simulink model "case8"  (R2024b)
settings: Solver=FixedStepAuto  StartTime=0  StopTime=1  FixedStep=1e-7  RelTol=1e-3
values from neighbouring files (symbols this model uses):
  SG_D_1_D = 0.01056    [IEEE9_case_parameters.m]    (also in case1_parameters.m; case2_parameters.m; case3_parameters.m; case4_parameters.m)
  SG_D_1_EnableSaturation = 0    [IEEE9_case_parameters.m]    (also in case1_parameters.m; case2_parameters.m; case3_parameters.m; case4_parameters.m)
  SG_D_1_f0 = 60    [IEEE9_case_parameters.m]    (also in case1_parameters.m; case2_parameters.m; case3_parameters.m; case4_parameters.m)
  SG_D_1_H = 7.5    [IEEE9_case_parameters.m]    (also in case1_parameters.m; case2_parameters.m; case3_parameters.m; case4_parameters.m)
  SG_D_1_K_A = 20    [IEEE9_case_parameters.m]    (also in case1_parameters.m; case2_parameters.m; case3_parameters.m; case4_parameters.m)
  SG_D_1_K_E = 1.000000e+1    (= 10)    [IEEE9_case_parameters.m]    (also in case1_parameters.m; case2_parameters.m; case3_parameters.m; case4_parameters.m)
  SG_D_1_K_F = 2.363    [IEEE9_case_parameters.m]    (also in case1_parameters.m; case2_parameters.m; case3_parameters.m; case4_parameters.m)
  SG_D_1_K_s = 0.5    [IEEE9_case_parameters.m]    (also in case1_parameters.m = 5; case2_parameters.m = 5; case3_parameters.m = 5; case4_parameters.m = 5)
  SG_D_1_R_a = 0.001088    [IEEE9_case_parameters.m]    (also in case1_parameters.m; case2_parameters.m; case3_parameters.m; case4_parameters.m)
  SG_D_1_S_A = 1    [IEEE9_case_parameters.m]    (also in case1_parameters.m; case2_parameters.m; case3_parameters.m; case4_parameters.m)
  SG_D_1_S_B = 0.103    [IEEE9_case_parameters.m]    (also in case1_parameters.m; case2_parameters.m; case3_parameters.m; case4_parameters.m)
  SG_D_1_S_N = 10.659857    [IEEE9_case_parameters.m]    (also in case1_parameters.m; case2_parameters.m; case3_parameters.m; case4_parameters.m)
  SG_D_1_SpeedPara = 200    [IEEE9_case_parameters.m]    (also in case1_parameters.m; case2_parameters.m; case3_parameters.m; case4_parameters.m)
  SG_D_1_T_0 = 0.720173    [IEEE9_case_parameters.m]    (also in case1_parameters.m = 0.755522; case2_parameters.m = 0.808931; case3_parameters.m = 0.869402; case4_parameters.m = 0.729316)
  SG_D_1_T_1 = 0.3    [IEEE9_case_parameters.m]    (also in case1_parameters.m; case2_parameters.m; case3_parameters.m; case4_parameters.m)
  SG_D_1_T_2 = 0.05    [IEEE9_case_parameters.m]    (also in case1_parameters.m; case2_parameters.m; case3_parameters.m; case4_parameters.m)
  SG_D_1_T_3 = 0.02    [IEEE9_case_parameters.m]    (also in case1_parameters.m; case2_parameters.m; case3_parameters.m; case4_parameters.m)
  SG_D_1_T_4 = 0.005    [IEEE9_case_parameters.m]    (also in case1_parameters.m; case2_parameters.m; case3_parameters.m; case4_parameters.m)
  SG_D_1_T_A = 0.02    [IEEE9_case_parameters.m]    (also in case1_parameters.m; case2_parameters.m; case3_parameters.m; case4_parameters.m)
  SG_D_1_T_dd = 8.000000e+0    (= 8)    [IEEE9_case_parameters.m]    (also in case1_parameters.m; case2_parameters.m; case3_parameters.m; case4_parameters.m)
  SG_D_1_T_ddd = 0.04    [IEEE9_case_parameters.m]    (also in case1_parameters.m; case2_parameters.m; case3_parameters.m; case4_parameters.m)
  SG_D_1_T_E = 0.314    [IEEE9_case_parameters.m]    (also in case1_parameters.m; case2_parameters.m; case3_parameters.m; case4_parameters.m)
  SG_D_1_T_F = 0.35    [IEEE9_case_parameters.m]    (also in case1_parameters.m; case2_parameters.m; case3_parameters.m; case4_parameters.m)
  SG_D_1_T_qd = 0.8    [IEEE9_case_parameters.m]    (also in case1_parameters.m; case2_parameters.m; case3_parameters.m; case4_parameters.m)
  SG_D_1_T_qdd = 0.02    [IEEE9_case_parameters.m]    (also in case1_parameters.m; case2_parameters.m; case3_parameters.m; case4_parameters.m)
  SG_D_1_T_speed = 0.1    [IEEE9_case_parameters.m]    (also in case1_parameters.m = 200; case2_parameters.m = 200; case3_parameters.m = 200; case4_parameters.m = 200)
  SG_D_1_T_w = 0.5    [IEEE9_case_parameters.m]    (also in case1_parameters.m; case2_parameters.m; case3_parameters.m; case4_parameters.m)
  SG_D_1_V_ref = 1.990276    [IEEE9_case_parameters.m]    (also in case1_parameters.m = 2.042296; case2_parameters.m = 2.051388; case3_parameters.m = 2.089584; case4_parameters.m = 2.01845)
  SG_D_1_w_ref = 376.991118    [IEEE9_case_parameters.m]    (also in case1_parameters.m; case2_parameters.m; case3_parameters.m; case4_parameters.m)
  SG_D_1_wb = 6.000000e+1    (= 60)    [IEEE9_case_parameters.m]    (also in case1_parameters.m; case2_parameters.m; case3_parameters.m; case4_parameters.m)
  SG_D_1_x_d = 1.9    [IEEE9_case_parameters.m]    (also in case1_parameters.m; case2_parameters.m; case3_parameters.m; case4_parameters.m)
  SG_D_1_x_dd = 0.302    [IEEE9_case_parameters.m]    (also in case1_parameters.m; case2_parameters.m; case3_parameters.m; case4_parameters.m)
  SG_D_1_x_ddd = 0.204    [IEEE9_case_parameters.m]    (also in case1_parameters.m; case2_parameters.m; case3_parameters.m; case4_parameters.m)
  SG_D_1_x_l = 0.05    [IEEE9_case_parameters.m]    (also in case1_parameters.m; case2_parameters.m; case3_parameters.m; case4_parameters.m)
  SG_D_1_x_q = 1.3    [IEEE9_case_parameters.m]    (also in case1_parameters.m; case2_parameters.m; case3_parameters.m; case4_parameters.m)
  SG_D_1_x_qd = 0.5    [IEEE9_case_parameters.m]    (also in case1_parameters.m; case2_parameters.m; case3_parameters.m; case4_parameters.m)
  SG_D_1_x_qdd = 0.3    [IEEE9_case_parameters.m]    (also in case1_parameters.m; case2_parameters.m; case3_parameters.m; case4_parameters.m)
  SG_D_2_D = 0.02    [IEEE9_case_parameters.m]    (also in case1_parameters.m; case2_parameters.m; case3_parameters.m; case4_parameters.m)
  SG_D_2_EnableSaturation = 0    [IEEE9_case_parameters.m]    (also in case1_parameters.m; case2_parameters.m; case3_parameters.m; case4_parameters.m)
  SG_D_2_f0 = 60    [IEEE9_case_parameters.m]    (also in case1_parameters.m; case2_parameters.m; case3_parameters.m; case4_parameters.m)
  SG_D_2_H = 8.000000e+0    (= 8)    [IEEE9_case_parameters.m]    (also in case1_parameters.m; case2_parameters.m; case3_parameters.m; case4_parameters.m)
  SG_D_2_K_A = 20    [IEEE9_case_parameters.m]    (also in case1_parameters.m; case2_parameters.m; case3_parameters.m; case4_parameters.m)
  SG_D_2_K_E = 1.000000e+1    (= 10)    [IEEE9_case_parameters.m]    (also in case1_parameters.m; case2_parameters.m; case3_parameters.m; case4_parameters.m)
  SG_D_2_K_F = 2.363    [IEEE9_case_parameters.m]    (also in case1_parameters.m; case2_parameters.m; case3_parameters.m; case4_parameters.m)
  SG_D_2_K_s = 0.5    [IEEE9_case_parameters.m]    (also in case1_parameters.m = 4; case2_parameters.m = 4; case3_parameters.m = 4; case4_parameters.m = 4)
  SG_D_2_R_a = 0.001088    [IEEE9_case_parameters.m]    (also in case1_parameters.m; case2_parameters.m; case3_parameters.m; case4_parameters.m)
  SG_D_2_S_A = 1    [IEEE9_case_parameters.m]    (also in case1_parameters.m; case2_parameters.m; case3_parameters.m; case4_parameters.m)
  SG_D_2_S_B = 0.103    [IEEE9_case_parameters.m]    (also in case1_parameters.m; case2_parameters.m; case3_parameters.m; case4_parameters.m)
  SG_D_2_S_N = 10.659857    [IEEE9_case_parameters.m]    (also in case1_parameters.m; case2_parameters.m; case3_parameters.m; case4_parameters.m)
  SG_D_2_SpeedPara = 200    [IEEE9_case_parameters.m]    (also in case1_parameters.m; case2_parameters.m; case3_parameters.m; case4_parameters.m)
  SG_D_2_T_0 = 1.632913    [IEEE9_case_parameters.m]    (also in case1_parameters.m = 1.632925; case2_parameters.m = 1.632915; case3_parameters.m = 1.632914; case4_parameters.m = 1.632927)
  SG_D_2_T_1 = 0.2    [IEEE9_case_parameters.m]    (also in case1_parameters.m; case2_parameters.m; case3_parameters.m; case4_parameters.m)
  SG_D_2_T_2 = 0.05    [IEEE9_case_parameters.m]    (also in case1_parameters.m; case2_parameters.m; case3_parameters.m; case4_parameters.m)
  SG_D_2_T_3 = 0.02    [IEEE9_case_parameters.m]    (also in case1_parameters.m; case2_parameters.m; case3_parameters.m; case4_parameters.m)
  SG_D_2_T_4 = 0.005    [IEEE9_case_parameters.m]    (also in case1_parameters.m; case2_parameters.m; case3_parameters.m; case4_parameters.m)
  SG_D_2_T_A = 0.02    [IEEE9_case_parameters.m]    (also in case1_parameters.m; case2_parameters.m; case3_parameters.m; case4_parameters.m)
  SG_D_2_T_dd = 7.9    [IEEE9_case_parameters.m]    (also in case1_parameters.m; case2_parameters.m; case3_parameters.m; case4_parameters.m)
  SG_D_2_T_ddd = 0.04    [IEEE9_case_parameters.m]    (also in case1_parameters.m; case2_parameters.m; case3_parameters.m; case4_parameters.m)
  SG_D_2_T_E = 0.314    [IEEE9_case_parameters.m]    (also in case1_parameters.m; case2_parameters.m; case3_parameters.m; case4_parameters.m)
  SG_D_2_T_F = 0.35    [IEEE9_case_parameters.m]    (also in case1_parameters.m; case2_parameters.m; case3_parameters.m; case4_parameters.m)
  SG_D_2_T_qd = 0.8    [IEEE9_case_parameters.m]    (also in case1_parameters.m; case2_parameters.m; case3_parameters.m; case4_parameters.m)
  SG_D_2_T_qdd = 0.015    [IEEE9_case_parameters.m]    (also in case1_parameters.m; case2_parameters.m; case3_parameters.m; case4_parameters.m)
  SG_D_2_T_speed = 0.1    [IEEE9_case_parameters.m]    (also in case1_parameters.m = 150; case2_parameters.m = 150; case3_parameters.m = 150; case4_parameters.m = 150)
  SG_D_2_T_w = 0.35    [IEEE9_case_parameters.m]    (also in case1_parameters.m; case2_parameters.m; case3_parameters.m; case4_parameters.m)
  SG_D_2_V_ref = 2.58547    [IEEE9_case_parameters.m]    (also in case1_parameters.m = 2.597896; case2_parameters.m = 2.587136; case3_parameters.m = 2.586042; case4_parameters.m = 2.599679)
  SG_D_2_w_ref = 376.991118    [IEEE9_case_parameters.m]    (also in case1_parameters.m; case2_parameters.m; case3_parameters.m; case4_parameters.m)
  SG_D_2_wb = 6.000000e+1    (= 60)    [IEEE9_case_parameters.m]    (also in case1_parameters.m; case2_parameters.m; case3_parameters.m; case4_parameters.m)
  SG_D_2_x_d = 1.8    [IEEE9_case_parameters.m]    (also in case1_parameters.m; case2_parameters.m; case3_parameters.m; case4_parameters.m)
  SG_D_2_x_dd = 0.302    [IEEE9_case_parameters.m]    (also in case1_parameters.m; case2_parameters.m; case3_parameters.m; case4_parameters.m)
  SG_D_2_x_ddd = 0.204    [IEEE9_case_parameters.m]    (also in case1_parameters.m; case2_parameters.m; case3_parameters.m; case4_parameters.m)
  SG_D_2_x_l = 0.05    [IEEE9_case_parameters.m]    (also in case1_parameters.m; case2_parameters.m; case3_parameters.m; case4_parameters.m)
  SG_D_2_x_q = 1.25    [IEEE9_case_parameters.m]    (also in case1_parameters.m; case2_parameters.m; case3_parameters.m; case4_parameters.m)
  SG_D_2_x_qd = 0.5    [IEEE9_case_parameters.m]    (also in case1_parameters.m; case2_parameters.m; case3_parameters.m; case4_parameters.m)
  SG_D_2_x_qdd = 0.3    [IEEE9_case_parameters.m]    (also in case1_parameters.m; case2_parameters.m; case3_parameters.m; case4_parameters.m)
  SG_D_3_D = 0.02    [IEEE9_case_parameters.m]    (also in case1_parameters.m; case2_parameters.m; case3_parameters.m; case4_parameters.m)
  SG_D_3_EnableSaturation = 0    [IEEE9_case_parameters.m]    (also in case1_parameters.m; case2_parameters.m; case3_parameters.m; case4_parameters.m)
  SG_D_3_f0 = 60    [IEEE9_case_parameters.m]    (also in case1_parameters.m; case2_parameters.m; case3_parameters.m; case4_parameters.m)
  SG_D_3_H = 7.7    [IEEE9_case_parameters.m]    (also in case1_parameters.m; case2_parameters.m; case3_parameters.m; case4_parameters.m)
  SG_D_3_K_A = 20    [IEEE9_case_parameters.m]    (also in case1_parameters.m; case2_parameters.m; case3_parameters.m; case4_parameters.m)
  SG_D_3_K_E = 1.000000e+1    (= 10)    [IEEE9_case_parameters.m]    (also in case1_parameters.m; case2_parameters.m; case3_parameters.m; case4_parameters.m)
  SG_D_3_K_F = 2.363    [IEEE9_case_parameters.m]    (also in case1_parameters.m; case2_parameters.m; case3_parameters.m; case4_parameters.m)
  SG_D_3_K_s = 0.2    [IEEE9_case_parameters.m]    (also in case1_parameters.m = 2; case2_parameters.m = 2; case3_parameters.m = 2; case4_parameters.m = 2)
  SG_D_3_R_a = 0.001088    [IEEE9_case_parameters.m]    (also in case1_parameters.m; case2_parameters.m; case3_parameters.m; case4_parameters.m)
  SG_D_3_S_A = 1    [IEEE9_case_parameters.m]    (also in case1_parameters.m; case2_parameters.m; case3_parameters.m; case4_parameters.m)
  SG_D_3_S_B = 0.103    [IEEE9_case_parameters.m]    (also in case1_parameters.m; case2_parameters.m; case3_parameters.m; case4_parameters.m)
  SG_D_3_S_N = 10.659857    [IEEE9_case_parameters.m]    (also in case1_parameters.m; case2_parameters.m; case3_parameters.m; case4_parameters.m)
  SG_D_3_SpeedPara = 200    [IEEE9_case_parameters.m]    (also in case1_parameters.m; case2_parameters.m; case3_parameters.m; case4_parameters.m)
  SG_D_3_T_0 = 0.850788    [IEEE9_case_parameters.m]    (also in case1_parameters.m = 0.850786; case2_parameters.m = 0.850787; case3_parameters.m; case4_parameters.m = 0.850786)
  SG_D_3_T_1 = 0.2    [IEEE9_case_parameters.m]    (also in case1_parameters.m; case2_parameters.m; case3_parameters.m; case4_parameters.m)
  SG_D_3_T_2 = 0.05    [IEEE9_case_parameters.m]    (also in case1_parameters.m; case2_parameters.m; case3_parameters.m; case4_parameters.m)
  SG_D_3_T_3 = 0.02    [IEEE9_case_parameters.m]    (also in case1_parameters.m; case2_parameters.m; case3_parameters.m; case4_parameters.m)
  SG_D_3_T_4 = 0.005    [IEEE9_case_parameters.m]    (also in case1_parameters.m; case2_parameters.m; case3_parameters.m; case4_parameters.m)
  SG_D_3_T_A = 0.02    [IEEE9_case_parameters.m]    (also in case1_parameters.m; case2_parameters.m; case3_parameters.m; case4_parameters.m)
  SG_D_3_T_dd = 8.1    [IEEE9_case_parameters.m]    (also in case1_parameters.m; case2_parameters.m; case3_parameters.m; case4_parameters.m)
  SG_D_3_T_ddd = 0.04    [IEEE9_case_parameters.m]    (also in case1_parameters.m; case2_parameters.m; case3_parameters.m; case4_parameters.m)
  SG_D_3_T_E = 0.314    [IEEE9_case_parameters.m]    (also in case1_parameters.m; case2_parameters.m; case3_parameters.m; case4_parameters.m)
  SG_D_3_T_F = 0.35    [IEEE9_case_parameters.m]    (also in case1_parameters.m; case2_parameters.m; case3_parameters.m; case4_parameters.m)
  SG_D_3_T_qd = 0.8    [IEEE9_case_parameters.m]    (also in case1_parameters.m; case2_parameters.m; case3_parameters.m; case4_parameters.m)
  SG_D_3_T_qdd = 0.015    [IEEE9_case_parameters.m]    (also in case1_parameters.m; case2_parameters.m; case3_parameters.m; case4_parameters.m)
  SG_D_3_T_speed = 0.1    [IEEE9_case_parameters.m]    (also in case1_parameters.m = 180; case2_parameters.m = 180; case3_parameters.m = 180; case4_parameters.m = 180)
  SG_D_3_T_w = 0.4    [IEEE9_case_parameters.m]    (also in case1_parameters.m; case2_parameters.m; case3_parameters.m; case4_parameters.m)
  SG_D_3_V_ref = 1.892727    [IEEE9_case_parameters.m]    (also in case1_parameters.m = 1.906439; case2_parameters.m = 1.895535; case3_parameters.m = 1.892105; case4_parameters.m = 1.906598)
  SG_D_3_w_ref = 376.991118    [IEEE9_case_parameters.m]    (also in case1_parameters.m; case2_parameters.m; case3_parameters.m; case4_parameters.m)
  SG_D_3_wb = 6.000000e+1    (= 60)    [IEEE9_case_parameters.m]    (also in case1_parameters.m; case2_parameters.m; case3_parameters.m; case4_parameters.m)
  SG_D_3_x_d = 1.85    [IEEE9_case_parameters.m]    (also in case1_parameters.m; case2_parameters.m; case3_parameters.m; case4_parameters.m)
  SG_D_3_x_dd = 0.302    [IEEE9_case_parameters.m]    (also in case1_parameters.m; case2_parameters.m; case3_parameters.m; case4_parameters.m)
  SG_D_3_x_ddd = 0.204    [IEEE9_case_parameters.m]    (also in case1_parameters.m; case2_parameters.m; case3_parameters.m; case4_parameters.m)
  SG_D_3_x_l = 0.05    [IEEE9_case_parameters.m]    (also in case1_parameters.m; case2_parameters.m; case3_parameters.m; case4_parameters.m)
  SG_D_3_x_q = 1.2    [IEEE9_case_parameters.m]    (also in case1_parameters.m; case2_parameters.m; case3_parameters.m; case4_parameters.m)
  SG_D_3_x_qd = 0.5    [IEEE9_case_parameters.m]    (also in case1_parameters.m; case2_parameters.m; case3_parameters.m; case4_parameters.m)
  SG_D_3_x_qdd = 0.3    [IEEE9_case_parameters.m]    (also in case1_parameters.m; case2_parameters.m; case3_parameters.m; case4_parameters.m)
(part 2 of 12)

== system case8/SG_D_2 ==
  v_d_SG_D_2 : Inport
  v_q_SG_D_2 : Inport  Port=2
  E_fd_SG_D_2 : Integrator  InitialCondition=3.1461551283845077
  Px_1_SG_D_2 : Integrator  InitialCondition=0.0
  Px_2_SG_D_2 : Integrator  InitialCondition=0.0
  Px_3_SG_D_2 : Integrator  InitialCondition=-1.4463668526796511e-25
  R_f_SG_D_2 : Integrator  InitialCondition=21.241041623921692
  T_e_SG_D_2_block : Subsystem
  T_m_SG_D_2 : Integrator  InitialCondition=1.6329038289025481
  V_f_SG_D_2 : Integrator  InitialCondition=31.46155128384508
  d_E_fd_SG_D_2_block : Subsystem
  d_Px_1_SG_D_2_block : Subsystem
  d_Px_2_SG_D_2_block : Subsystem
  d_Px_3_SG_D_2_block : Subsystem
  d_R_f_SG_D_2_block : Subsystem
  d_T_m_SG_D_2_block : Subsystem
  d_V_f_SG_D_2_block : Subsystem
  d_psi_1d_SG_D_2_block : Subsystem
  d_psi_d_SG_D_2_block : Subsystem
  d_psi_fd_SG_D_2_block : Subsystem
  d_psi_gq_SG_D_2_block : Subsystem
  d_psi_kq_SG_D_2_block : Subsystem
  d_psi_q_SG_D_2_block : Subsystem
  d_theta_SG_D_2_block : Subsystem
  d_w_SG_D_2_block : Subsystem
  i_d_SG_D_2_block : Subsystem
  i_q_SG_D_2_block : Subsystem
  psi_1d_SG_D_2 : Integrator  InitialCondition=0.5625664495240386
  psi_d_SG_D_2 : Integrator  InitialCondition=0.4887496301280251
  psi_fd_SG_D_2 : Integrator  InitialCondition=0.9346032192799462
  psi_gq_SG_D_2 : Integrator  InitialCondition=0.524673786109037
  psi_kq_SG_D_2 : Integrator  InitialCondition=-0.8394780577744592
  psi_q_SG_D_2 : Integrator  InitialCondition=-0.8744563101817284
  theta_SG_D_2 : Integrator  InitialCondition=1.2359602856549958
  theta_SG_D_2_out_block : Subsystem
  w_SG_D_2 : Integrator  InitialCondition=376.99111843077515
  w_SG_D_2_out_block : Subsystem
  i_d_SG_D_2 : Outport
  i_q_SG_D_2 : Outport  Port=2
  T_e_SG_D_2 : Outport  Port=3
  w_SG_D_2_out : Outport  Port=4
  theta_SG_D_2_out : Outport  Port=5
  wires:
  T_e_SG_D_2_block/1(Blockout_T_e_SG_D_2_37eed) -> T_e_SG_D_2/1
  d_Px_2_SG_D_2_block/1(Blockout_d_Px_2_SG_D_2_834a7) -> Px_2_SG_D_2/1
  d_T_m_SG_D_2_block/1(Blockout_d_T_m_SG_D_2_9d432) -> T_m_SG_D_2/1
  w_SG_D_2/1 -> d_psi_d_SG_D_2_block/9(State_w_SG_D_2_45274), d_psi_q_SG_D_2_block/9(State_w_SG_D_2_341ca), d_w_SG_D_2_block/1(State_w_SG_D_2_ba66f), d_V_f_SG_D_2_block/8(State_w_SG_D_2_40010), d_V_f_SG_D_2_block/13(State_w_SG_D_2_e6aa6), d_T_m_SG_D_2_block/1(State_w_SG_D_2_f6fcd), d_Px_1_SG_D_2_block/2(State_w_SG_D_2_e8896), d_Px_2_SG_D_2_block/4(State_w_SG_D_2_770a4), d_theta_SG_D_2_block/1(State_w_SG_D_2_7bd31), d_Px_3_SG_D_2_block/6(State_w_SG_D_2_e0f2c), w_SG_D_2_out_block/1(State_w_SG_D_2_c1838)
  psi_fd_SG_D_2/1 -> d_psi_fd_SG_D_2_block/4(State_psi_fd_SG_D_2_4158a), d_psi_fd_SG_D_2_block/2(State_psi_fd_SG_D_2_b4c0c), d_psi_fd_SG_D_2_block/7(State_psi_fd_SG_D_2_07a98), d_psi_fd_SG_D_2_block/10(State_psi_fd_SG_D_2_1b762), d_psi_d_SG_D_2_block/3(State_psi_fd_SG_D_2_72f19), d_psi_1d_SG_D_2_block/2(State_psi_fd_SG_D_2_ceb12), d_psi_1d_SG_D_2_block/5(State_psi_fd_SG_D_2_a1da1), i_d_SG_D_2_block/7(State_psi_fd_SG_D_2_bfe7a), i_q_SG_D_2_block/7(State_psi_fd_SG_D_2_88a91), d_w_SG_D_2_block/10(State_psi_fd_SG_D_2_18877), d_V_f_SG_D_2_block/6(State_psi_fd_SG_D_2_2a738), T_e_SG_D_2_block/8(State_psi_fd_SG_D_2_89a99)
  d_Px_3_SG_D_2_block/1(Blockout_d_Px_3_SG_D_2_f4998) -> Px_3_SG_D_2/1
  d_theta_SG_D_2_block/1(Blockout_d_theta_SG_D_2_25192) -> theta_SG_D_2/1
  psi_q_SG_D_2/1 -> d_psi_d_SG_D_2_block/8(State_psi_q_SG_D_2_6ca96), d_psi_q_SG_D_2_block/3(State_psi_q_SG_D_2_4fbbc), d_psi_gq_SG_D_2_block/6(State_psi_q_SG_D_2_7c5c2), d_psi_gq_SG_D_2_block/9(State_psi_q_SG_D_2_071fc), d_psi_kq_SG_D_2_block/5(State_psi_q_SG_D_2_e3912), d_w_SG_D_2_block/6(State_psi_q_SG_D_2_719d4), d_V_f_SG_D_2_block/7(State_psi_q_SG_D_2_06b5a), d_w_SG_D_2_block/7(State_psi_q_SG_D_2_47440), d_V_f_SG_D_2_block/11(State_psi_q_SG_D_2_14190), T_e_SG_D_2_block/4(State_psi_q_SG_D_2_d1f35), i_d_SG_D_2_block/3(State_psi_q_SG_D_2_62810), T_e_SG_D_2_block/5(State_psi_q_SG_D_2_dcfde), i_q_SG_D_2_block/3(State_psi_q_SG_D_2_6a090)
  w_SG_D_2_out_block/1(Blockout_w_SG_D_2_out_5dbba) -> w_SG_D_2_out/1
  d_Px_1_SG_D_2_block/1(Blockout_d_Px_1_SG_D_2_3d98f) -> Px_1_SG_D_2/1
  theta_SG_D_2/1 -> d_psi_d_SG_D_2_block/5(State_theta_SG_D_2_93d8b), d_psi_d_SG_D_2_block/7(State_theta_SG_D_2_1c678), d_psi_q_SG_D_2_block/7(State_theta_SG_D_2_47452), i_d_SG_D_2_block/4(State_theta_SG_D_2_8321e), i_q_SG_D_2_block/4(State_theta_SG_D_2_61b92), i_q_SG_D_2_block/8(State_theta_SG_D_2_36c34), i_d_SG_D_2_block/8(State_theta_SG_D_2_8d67b), theta_SG_D_2_out_block/1(State_theta_SG_D_2_588b5), d_psi_q_SG_D_2_block/5(State_theta_SG_D_2_e72a3)
  v_d_SG_D_2/1 -> d_psi_d_SG_D_2_block/4(Input_v_d_SG_D_2_0b52f), d_psi_q_SG_D_2_block/4(Input_v_d_SG_D_2_d12f5)
  psi_gq_SG_D_2/1 -> d_psi_q_SG_D_2_block/1(State_psi_gq_SG_D_2_5ef83), d_psi_gq_SG_D_2_block/1(State_psi_gq_SG_D_2_6e627), d_psi_gq_SG_D_2_block/2(State_psi_gq_SG_D_2_262b6), d_psi_gq_SG_D_2_block/4(State_psi_gq_SG_D_2_5c0ba), d_psi_kq_SG_D_2_block/3(State_psi_gq_SG_D_2_5efea), d_w_SG_D_2_block/4(State_psi_gq_SG_D_2_4cbe9), d_psi_gq_SG_D_2_block/7(State_psi_gq_SG_D_2_708e2), d_V_f_SG_D_2_block/9(State_psi_gq_SG_D_2_0beb3), d_psi_kq_SG_D_2_block/1(State_psi_gq_SG_D_2_71331), T_e_SG_D_2_block/2(State_psi_gq_SG_D_2_6b895), i_q_SG_D_2_block/1(State_psi_gq_SG_D_2_ca4a4), i_d_SG_D_2_block/1(State_psi_gq_SG_D_2_6632a)
  d_V_f_SG_D_2_block/1(Blockout_d_V_f_SG_D_2_ff4c4) -> V_f_SG_D_2/1
  v_q_SG_D_2/1 -> d_psi_d_SG_D_2_block/6(Input_v_q_SG_D_2_24264), d_psi_q_SG_D_2_block/6(Input_v_q_SG_D_2_08eca)
  psi_kq_SG_D_2/1 -> d_psi_q_SG_D_2_block/2(State_psi_kq_SG_D_2_f0515), d_psi_gq_SG_D_2_block/3(State_psi_kq_SG_D_2_70141), d_psi_gq_SG_D_2_block/5(State_psi_kq_SG_D_2_f72a7), d_psi_gq_SG_D_2_block/8(State_psi_kq_SG_D_2_8a990), d_w_SG_D_2_block/5(State_psi_kq_SG_D_2_af1ac), d_V_f_SG_D_2_block/10(State_psi_kq_SG_D_2_49fef), d_psi_kq_SG_D_2_block/2(State_psi_kq_SG_D_2_cb04f), i_d_SG_D_2_block/2(State_psi_kq_SG_D_2_999f9), i_q_SG_D_2_block/2(State_psi_kq_SG_D_2_2a403), T_e_SG_D_2_block/3(State_psi_kq_SG_D_2_20085), d_psi_kq_SG_D_2_block/4(State_psi_kq_SG_D_2_ff070)
  i_d_SG_D_2_block/1(Blockout_i_d_SG_D_2_06834) -> i_d_SG_D_2/1
  psi_d_SG_D_2/1 -> d_psi_fd_SG_D_2_block/9(State_psi_d_SG_D_2_0ff1e), d_psi_q_SG_D_2_block/8(State_psi_d_SG_D_2_64c51), d_psi_1d_SG_D_2_block/4(State_psi_d_SG_D_2_bd43f), d_w_SG_D_2_block/3(State_psi_d_SG_D_2_74fc0), d_psi_d_SG_D_2_block/2(State_psi_d_SG_D_2_6f046), d_psi_fd_SG_D_2_block/6(State_psi_d_SG_D_2_db85c), d_w_SG_D_2_block/9(State_psi_d_SG_D_2_c6663), d_V_f_SG_D_2_block/12(State_psi_d_SG_D_2_55d30), d_V_f_SG_D_2_block/5(State_psi_d_SG_D_2_02653), i_d_SG_D_2_block/6(State_psi_d_SG_D_2_05ecc), i_q_SG_D_2_block/6(State_psi_d_SG_D_2_04a53), T_e_SG_D_2_block/1(State_psi_d_SG_D_2_f5fd7), T_e_SG_D_2_block/7(State_psi_d_SG_D_2_0c163)
  Px_1_SG_D_2/1 -> d_Px_1_SG_D_2_block/1(State_Px_1_SG_D_2_1fdac), d_Px_2_SG_D_2_block/3(State_Px_1_SG_D_2_2790d), d_Px_3_SG_D_2_block/4(State_Px_1_SG_D_2_7fb84), d_Px_3_SG_D_2_block/5(State_Px_1_SG_D_2_3fef0), d_Px_2_SG_D_2_block/2(State_Px_1_SG_D_2_d6347)
  T_m_SG_D_2/1 -> d_T_m_SG_D_2_block/2(State_T_m_SG_D_2_95b0e), d_w_SG_D_2_block/2(State_T_m_SG_D_2_44cee)
  Px_2_SG_D_2/1 -> d_Px_2_SG_D_2_block/1(State_Px_2_SG_D_2_8f0fc), d_Px_3_SG_D_2_block/2(State_Px_2_SG_D_2_e8830), d_Px_3_SG_D_2_block/3(State_Px_2_SG_D_2_b92ad)
  psi_1d_SG_D_2/1 -> d_psi_fd_SG_D_2_block/8(State_psi_1d_SG_D_2_d512d), d_psi_fd_SG_D_2_block/5(State_psi_1d_SG_D_2_923e8), d_psi_d_SG_D_2_block/1(State_psi_1d_SG_D_2_aad77), d_psi_fd_SG_D_2_block/3(State_psi_1d_SG_D_2_30ef8), d_psi_1d_SG_D_2_block/3(State_psi_1d_SG_D_2_f87fc), d_w_SG_D_2_block/8(State_psi_1d_SG_D_2_235de), d_psi_1d_SG_D_2_block/1(State_psi_1d_SG_D_2_34802), d_V_f_SG_D_2_block/4(State_psi_1d_SG_D_2_6ad6a), i_d_SG_D_2_block/5(State_psi_1d_SG_D_2_4ff2d), i_q_SG_D_2_block/5(State_psi_1d_SG_D_2_1de77), T_e_SG_D_2_block/6(State_psi_1d_SG_D_2_b2612)
  d_R_f_SG_D_2_block/1(Blockout_d_R_f_SG_D_2_8501b) -> R_f_SG_D_2/1
  d_psi_gq_SG_D_2_block/1(Blockout_d_psi_gq_SG_D_2_9dda3) -> psi_gq_SG_D_2/1
  d_psi_kq_SG_D_2_block/1(Blockout_d_psi_kq_SG_D_2_314e9) -> psi_kq_SG_D_2/1
  R_f_SG_D_2/1 -> d_V_f_SG_D_2_block/2(State_R_f_SG_D_2_4eb2e), d_R_f_SG_D_2_block/2(State_R_f_SG_D_2_76268)
  theta_SG_D_2_out_block/1(Blockout_theta_SG_D_2_out_80a64) -> theta_SG_D_2_out/1
  i_q_SG_D_2_block/1(Blockout_i_q_SG_D_2_51e7b) -> i_q_SG_D_2/1
  d_psi_q_SG_D_2_block/1(Blockout_d_psi_q_SG_D_2_ca292) -> psi_q_SG_D_2/1
  d_psi_d_SG_D_2_block/1(Blockout_d_psi_d_SG_D_2_41311) -> psi_d_SG_D_2/1
  d_w_SG_D_2_block/1(Blockout_d_w_SG_D_2_560c9) -> w_SG_D_2/1
  d_psi_1d_SG_D_2_block/1(Blockout_d_psi_1d_SG_D_2_8d877) -> psi_1d_SG_D_2/1
  V_f_SG_D_2/1 -> d_V_f_SG_D_2_block/14(State_V_f_SG_D_2_79586), d_E_fd_SG_D_2_block/2(State_V_f_SG_D_2_b3f2e)
  Px_3_SG_D_2/1 -> d_V_f_SG_D_2_block/3(State_Px_3_SG_D_2_61526), d_Px_3_SG_D_2_block/1(State_Px_3_SG_D_2_a00f9)
  d_E_fd_SG_D_2_block/1(Blockout_d_E_fd_SG_D_2_a4411) -> E_fd_SG_D_2/1
  E_fd_SG_D_2/1 -> d_R_f_SG_D_2_block/1(State_E_fd_SG_D_2_59077), d_V_f_SG_D_2_block/1(State_E_fd_SG_D_2_d52e1), d_E_fd_SG_D_2_block/1(State_E_fd_SG_D_2_423a9), d_psi_fd_SG_D_2_block/1(State_E_fd_SG_D_2_e61ef)
  d_psi_fd_SG_D_2_block/1(Blockout_d_psi_fd_SG_D_2_e5dbf) -> psi_fd_SG_D_2/1

== system case8/SG_D_3 ==
  v_d_SG_D_3 : Inport
  v_q_SG_D_3 : Inport  Port=2
  E_fd_SG_D_3 : Integrator  InitialCondition=1.7532139531153585
  Px_1_SG_D_3 : Integrator  InitialCondition=0.0
  Px_2_SG_D_3 : Integrator  InitialCondition=0.0
  Px_3_SG_D_3 : Integrator  InitialCondition=9.861433339358398e-25
  R_f_SG_D_3 : Integrator  InitialCondition=11.836698774890264
  T_e_SG_D_3_block : Subsystem
  T_m_SG_D_3 : Integrator  InitialCondition=0.8507912366770715
  V_f_SG_D_3 : Integrator  InitialCondition=17.532139531153582
  d_E_fd_SG_D_3_block : Subsystem
  d_Px_1_SG_D_3_block : Subsystem
  d_Px_2_SG_D_3_block : Subsystem
  d_Px_3_SG_D_3_block : Subsystem
  d_R_f_SG_D_3_block : Subsystem
  d_T_m_SG_D_3_block : Subsystem
  d_V_f_SG_D_3_block : Subsystem
  d_psi_1d_SG_D_3_block : Subsystem
  d_psi_d_SG_D_3_block : Subsystem
  d_psi_fd_SG_D_3_block : Subsystem
  d_psi_gq_SG_D_3_block : Subsystem
  d_psi_kq_SG_D_3_block : Subsystem
  d_psi_q_SG_D_3_block : Subsystem
  d_theta_SG_D_3_block : Subsystem
  d_w_SG_D_3_block : Subsystem
  i_d_SG_D_3_block : Subsystem
  i_q_SG_D_3_block : Subsystem
  psi_1d_SG_D_3 : Integrator  InitialCondition=0.6990200101655261
  psi_d_SG_D_3 : Integrator  InitialCondition=0.6697368450835861
  psi_fd_SG_D_3 : Integrator  InitialCondition=0.8466071621785026
  psi_gq_SG_D_3 : Integrator  InitialCondition=0.4339086560646932
  psi_kq_SG_D_3 : Integrator  InitialCondition=-0.7128499349634246
  psi_q_SG_D_3 : Integrator  InitialCondition=-0.7438434103966169
  theta_SG_D_3 : Integrator  InitialCondition=0.9265669299712972
  theta_SG_D_3_out_block : Subsystem
  w_SG_D_3 : Integrator  InitialCondition=376.99111843077515
  w_SG_D_3_out_block : Subsystem
  i_d_SG_D_3 : Outport
  i_q_SG_D_3 : Outport  Port=2
  T_e_SG_D_3 : Outport  Port=3
  w_SG_D_3_out : Outport  Port=4
  theta_SG_D_3_out : Outport  Port=5
  wires:
  psi_q_SG_D_3/1 -> d_psi_d_SG_D_3_block/8(State_psi_q_SG_D_3_c42a8), d_psi_q_SG_D_3_block/3(State_psi_q_SG_D_3_c2b51), d_psi_gq_SG_D_3_block/6(State_psi_q_SG_D_3_5b7d5), d_psi_gq_SG_D_3_block/9(State_psi_q_SG_D_3_a2ccc), d_psi_kq_SG_D_3_block/5(State_psi_q_SG_D_3_9bd31), d_w_SG_D_3_block/6(State_psi_q_SG_D_3_ce2ac), d_V_f_SG_D_3_block/7(State_psi_q_SG_D_3_86bf4), d_w_SG_D_3_block/7(State_psi_q_SG_D_3_ecc92), i_d_SG_D_3_block/3(State_psi_q_SG_D_3_5ee11), T_e_SG_D_3_block/4(State_psi_q_SG_D_3_35d7e), i_q_SG_D_3_block/3(State_psi_q_SG_D_3_862db), T_e_SG_D_3_block/5(State_psi_q_SG_D_3_c727a), d_V_f_SG_D_3_block/11(State_psi_q_SG_D_3_c4568)
  d_Px_1_SG_D_3_block/1(Blockout_d_Px_1_SG_D_3_077a4) -> Px_1_SG_D_3/1
  w_SG_D_3/1 -> d_psi_q_SG_D_3_block/9(State_w_SG_D_3_cea80), d_w_SG_D_3_block/1(State_w_SG_D_3_f0746), d_V_f_SG_D_3_block/13(State_w_SG_D_3_9dc31), d_V_f_SG_D_3_block/8(State_w_SG_D_3_db882), d_psi_d_SG_D_3_block/9(State_w_SG_D_3_47940), d_theta_SG_D_3_block/1(State_w_SG_D_3_084e9), d_T_m_SG_D_3_block/1(State_w_SG_D_3_a06af), d_Px_2_SG_D_3_block/4(State_w_SG_D_3_f6faf), d_Px_3_SG_D_3_block/6(State_w_SG_D_3_68c48), w_SG_D_3_out_block/1(State_w_SG_D_3_ff000), d_Px_1_SG_D_3_block/2(State_w_SG_D_3_d97b7)
  d_Px_2_SG_D_3_block/1(Blockout_d_Px_2_SG_D_3_2ce39) -> Px_2_SG_D_3/1
  R_f_SG_D_3/1 -> d_V_f_SG_D_3_block/2(State_R_f_SG_D_3_115cf), d_R_f_SG_D_3_block/2(State_R_f_SG_D_3_58aed)
  w_SG_D_3_out_block/1(Blockout_w_SG_D_3_out_f99ae) -> w_SG_D_3_out/1
  d_Px_3_SG_D_3_block/1(Blockout_d_Px_3_SG_D_3_3c603) -> Px_3_SG_D_3/1
  d_T_m_SG_D_3_block/1(Blockout_d_T_m_SG_D_3_869a6) -> T_m_SG_D_3/1
  d_w_SG_D_3_block/1(Blockout_d_w_SG_D_3_79f11) -> w_SG_D_3/1
  Px_1_SG_D_3/1 -> d_Px_2_SG_D_3_block/2(State_Px_1_SG_D_3_29485), d_Px_3_SG_D_3_block/4(State_Px_1_SG_D_3_e800f), d_Px_3_SG_D_3_block/5(State_Px_1_SG_D_3_b0515), d_Px_1_SG_D_3_block/1(State_Px_1_SG_D_3_05451), d_Px_2_SG_D_3_block/3(State_Px_1_SG_D_3_7b549)
  d_theta_SG_D_3_block/1(Blockout_d_theta_SG_D_3_e0920) -> theta_SG_D_3/1
  psi_d_SG_D_3/1 -> d_psi_fd_SG_D_3_block/6(State_psi_d_SG_D_3_275f4), d_psi_fd_SG_D_3_block/9(State_psi_d_SG_D_3_8cb70), d_psi_q_SG_D_3_block/8(State_psi_d_SG_D_3_3d93d), d_psi_1d_SG_D_3_block/4(State_psi_d_SG_D_3_558ca), d_w_SG_D_3_block/9(State_psi_d_SG_D_3_30888), d_V_f_SG_D_3_block/5(State_psi_d_SG_D_3_a5146), d_V_f_SG_D_3_block/12(State_psi_d_SG_D_3_4db12), i_d_SG_D_3_block/6(State_psi_d_SG_D_3_2ac54), d_psi_d_SG_D_3_block/2(State_psi_d_SG_D_3_63877), d_w_SG_D_3_block/3(State_psi_d_SG_D_3_be5ef), i_q_SG_D_3_block/6(State_psi_d_SG_D_3_c33e0), T_e_SG_D_3_block/1(State_psi_d_SG_D_3_f2f0a), T_e_SG_D_3_block/7(State_psi_d_SG_D_3_7037a)
  psi_kq_SG_D_3/1 -> d_psi_q_SG_D_3_block/2(State_psi_kq_SG_D_3_afd1f), d_psi_gq_SG_D_3_block/3(State_psi_kq_SG_D_3_0d0cf), d_psi_gq_SG_D_3_block/5(State_psi_kq_SG_D_3_6a61a), d_psi_kq_SG_D_3_block/2(State_psi_kq_SG_D_3_44aa7), d_psi_gq_SG_D_3_block/8(State_psi_kq_SG_D_3_6c9a2), d_V_f_SG_D_3_block/10(State_psi_kq_SG_D_3_35249), d_psi_kq_SG_D_3_block/4(State_psi_kq_SG_D_3_0268c), i_d_SG_D_3_block/2(State_psi_kq_SG_D_3_4b8d1), i_q_SG_D_3_block/2(State_psi_kq_SG_D_3_44924), d_w_SG_D_3_block/5(State_psi_kq_SG_D_3_352ae), T_e_SG_D_3_block/3(State_psi_kq_SG_D_3_d23e5)
  d_psi_kq_SG_D_3_block/1(Blockout_d_psi_kq_SG_D_3_6329c) -> psi_kq_SG_D_3/1
  psi_1d_SG_D_3/1 -> d_psi_fd_SG_D_3_block/3(State_psi_1d_SG_D_3_ed615), d_psi_fd_SG_D_3_block/5(State_psi_1d_SG_D_3_498fb), d_psi_fd_SG_D_3_block/8(State_psi_1d_SG_D_3_b1cc2), d_psi_d_SG_D_3_block/1(State_psi_1d_SG_D_3_4ea1a), d_psi_1d_SG_D_3_block/3(State_psi_1d_SG_D_3_8c42f), d_w_SG_D_3_block/8(State_psi_1d_SG_D_3_4c859), d_V_f_SG_D_3_block/4(State_psi_1d_SG_D_3_782b3), i_d_SG_D_3_block/5(State_psi_1d_SG_D_3_83346), i_q_SG_D_3_block/5(State_psi_1d_SG_D_3_2f07b), T_e_SG_D_3_block/6(State_psi_1d_SG_D_3_3c424), d_psi_1d_SG_D_3_block/1(State_psi_1d_SG_D_3_f33a6)
  T_m_SG_D_3/1 -> d_T_m_SG_D_3_block/2(State_T_m_SG_D_3_22a90), d_w_SG_D_3_block/2(State_T_m_SG_D_3_db088)
  theta_SG_D_3/1 -> d_psi_d_SG_D_3_block/5(State_theta_SG_D_3_df685), i_d_SG_D_3_block/8(State_theta_SG_D_3_d9be7), i_d_SG_D_3_block/4(State_theta_SG_D_3_341cf), d_psi_d_SG_D_3_block/7(State_theta_SG_D_3_0fee2), i_q_SG_D_3_block/4(State_theta_SG_D_3_dfac9), d_psi_q_SG_D_3_block/5(State_theta_SG_D_3_3c006), i_q_SG_D_3_block/8(State_theta_SG_D_3_7932a), theta_SG_D_3_out_block/1(State_theta_SG_D_3_013d5), d_psi_q_SG_D_3_block/7(State_theta_SG_D_3_65b3a)
  v_d_SG_D_3/1 -> d_psi_d_SG_D_3_block/4(Input_v_d_SG_D_3_0c684), d_psi_q_SG_D_3_block/4(Input_v_d_SG_D_3_a1afd)
  v_q_SG_D_3/1 -> d_psi_d_SG_D_3_block/6(Input_v_q_SG_D_3_4be76), d_psi_q_SG_D_3_block/6(Input_v_q_SG_D_3_3c190)
  Px_2_SG_D_3/1 -> d_Px_2_SG_D_3_block/1(State_Px_2_SG_D_3_6d3a4), d_Px_3_SG_D_3_block/2(State_Px_2_SG_D_3_61442), d_Px_3_SG_D_3_block/3(State_Px_2_SG_D_3_31d74)
  psi_gq_SG_D_3/1 -> d_psi_q_SG_D_3_block/1(State_psi_gq_SG_D_3_bc5a9), d_psi_gq_SG_D_3_block/1(State_psi_gq_SG_D_3_1cd63), d_psi_gq_SG_D_3_block/2(State_psi_gq_SG_D_3_d752b), d_psi_gq_SG_D_3_block/4(State_psi_gq_SG_D_3_b078d), d_psi_gq_SG_D_3_block/7(State_psi_gq_SG_D_3_c8dd2), d_w_SG_D_3_block/4(State_psi_gq_SG_D_3_be34d), d_V_f_SG_D_3_block/9(State_psi_gq_SG_D_3_96b70), d_psi_kq_SG_D_3_block/3(State_psi_gq_SG_D_3_6d3fb), i_d_SG_D_3_block/1(State_psi_gq_SG_D_3_8b9f6), d_psi_kq_SG_D_3_block/1(State_psi_gq_SG_D_3_1d67a), i_q_SG_D_3_block/1(State_psi_gq_SG_D_3_60a8f), T_e_SG_D_3_block/2(State_psi_gq_SG_D_3_975c9)
  psi_fd_SG_D_3/1 -> d_psi_fd_SG_D_3_block/4(State_psi_fd_SG_D_3_b9793), d_psi_fd_SG_D_3_block/7(State_psi_fd_SG_D_3_7365a), d_psi_fd_SG_D_3_block/10(State_psi_fd_SG_D_3_47206), d_psi_fd_SG_D_3_block/2(State_psi_fd_SG_D_3_191f5), d_psi_d_SG_D_3_block/3(State_psi_fd_SG_D_3_636d2), d_psi_1d_SG_D_3_block/5(State_psi_fd_SG_D_3_d2e28), d_V_f_SG_D_3_block/6(State_psi_fd_SG_D_3_73ebf), d_w_SG_D_3_block/10(State_psi_fd_SG_D_3_e9214), d_psi_1d_SG_D_3_block/2(State_psi_fd_SG_D_3_35873), i_q_SG_D_3_block/7(State_psi_fd_SG_D_3_a451c), T_e_SG_D_3_block/8(State_psi_fd_SG_D_3_db5f7), i_d_SG_D_3_block/7(State_psi_fd_SG_D_3_bd64a)
  d_psi_q_SG_D_3_block/1(Blockout_d_psi_q_SG_D_3_2b12b) -> psi_q_SG_D_3/1
  d_R_f_SG_D_3_block/1(Blockout_d_R_f_SG_D_3_82a7f) -> R_f_SG_D_3/1
  theta_SG_D_3_out_block/1(Blockout_theta_SG_D_3_out_8d530) -> theta_SG_D_3_out/1
  d_V_f_SG_D_3_block/1(Blockout_d_V_f_SG_D_3_a30cd) -> V_f_SG_D_3/1
  T_e_SG_D_3_block/1(Blockout_T_e_SG_D_3_28e2c) -> T_e_SG_D_3/1
  d_psi_1d_SG_D_3_block/1(Blockout_d_psi_1d_SG_D_3_b77c8) -> psi_1d_SG_D_3/1
  d_psi_d_SG_D_3_block/1(Blockout_d_psi_d_SG_D_3_3f46c) -> psi_d_SG_D_3/1
  i_d_SG_D_3_block/1(Blockout_i_d_SG_D_3_d7069) -> i_d_SG_D_3/1
  i_q_SG_D_3_block/1(Blockout_i_q_SG_D_3_b1dd0) -> i_q_SG_D_3/1
  d_psi_gq_SG_D_3_block/1(Blockout_d_psi_gq_SG_D_3_df242) -> psi_gq_SG_D_3/1
  V_f_SG_D_3/1 -> d_V_f_SG_D_3_block/14(State_V_f_SG_D_3_de5b8), d_E_fd_SG_D_3_block/2(State_V_f_SG_D_3_cf6c5)
  Px_3_SG_D_3/1 -> d_V_f_SG_D_3_block/3(State_Px_3_SG_D_3_e0d4b), d_Px_3_SG_D_3_block/1(State_Px_3_SG_D_3_01303)
  d_E_fd_SG_D_3_block/1(Blockout_d_E_fd_SG_D_3_7634c) -> E_fd_SG_D_3/1
  E_fd_SG_D_3/1 -> d_V_f_SG_D_3_block/1(State_E_fd_SG_D_3_5e56b), d_R_f_SG_D_3_block/1(State_E_fd_SG_D_3_84f8d), d_E_fd_SG_D_3_block/1(State_E_fd_SG_D_3_3a99a), d_psi_fd_SG_D_3_block/1(State_E_fd_SG_D_3_14ff0)
  d_psi_fd_SG_D_3_block/1(Blockout_d_psi_fd_SG_D_3_efa73) -> psi_fd_SG_D_3/1

== system case8/AC_1/d_id_line_1_4_block ==
  note: d_id_line_1_4 in case8
      | $376.991118430775\,\mathrm{iq}_{\mathrm{line},1,4}+6464.71823947318\,\mathrm{vd}_{\mathrm{bus},1}-6464.71823947318\,\mathrm{vd}_{\mathrm{bus},4}$
      | Automatically generated on 2025-10-31 19:30:31 .
  State_iq_line_1_4_fbe14 : Inport
  State_vd_bus_1_49433 : Inport  Port=2
  State_vd_bus_4_56409 : Inport  Port=3
  Add_c41cb : Sum
  Constant_376.991118430775_c4186 : Constant  Value=376.991118430775
  Constant_6464.71823947318_799c5 : Constant  Value=6464.71823947318
  Constant_6464.71823947318_82374 : Constant  Value=6464.71823947318
  Product_20401 : Product
  Product_ed597 : Product
  Product_f78cd : Product
  Subtract_ed0f5 : Sum  Inputs=+-
  Blockout_d_id_line_1_4_ee914 : Outport
  wires:
  Constant_376.991118430775_c4186/1 -> Product_f78cd/1
  Product_20401/1 -> Add_c41cb/2
  State_iq_line_1_4_fbe14/1 -> Product_f78cd/2
  Subtract_ed0f5/1 -> Blockout_d_id_line_1_4_ee914/1
  Constant_6464.71823947318_799c5/1 -> Product_20401/1
  Product_f78cd/1 -> Add_c41cb/1
  State_vd_bus_1_49433/1 -> Product_20401/2
  Constant_6464.71823947318_82374/1 -> Product_ed597/1
  State_vd_bus_4_56409/1 -> Product_ed597/2
  Add_c41cb/1 -> Subtract_ed0f5/1
  Product_ed597/1 -> Subtract_ed0f5/2

== system case8/AC_1/d_id_line_3_6_block ==
  note: d_id_line_3_6 in case8
      | $376.991118430775\,\mathrm{iq}_{\mathrm{line},3,6}+6354.39881559139\,\mathrm{vd}_{\mathrm{bus},3}-6354.39881559139\,\mathrm{vd}_{\mathrm{bus},6}$
      | Automatically generated on 2025-10-31 19:30:34 .
  State_iq_line_3_6_a71b0 : Inport
  State_vd_bus_3_123b1 : Inport  Port=2
  State_vd_bus_6_bb3d9 : Inport  Port=3
  Add_49cf9 : Sum
  Constant_376.991118430775_75d3f : Constant  Value=376.991118430775
  Constant_6354.39881559139_a08a5 : Constant  Value=6354.39881559139
  Constant_6354.39881559139_fd121 : Constant  Value=6354.39881559139
  Product_0c19c : Product
  Product_c7c72 : Product
  Product_cb8fd : Product
  Subtract_b6367 : Sum  Inputs=+-
  Blockout_d_id_line_3_6_73b84 : Outport
  wires:
  State_vd_bus_3_123b1/1 -> Product_c7c72/2
  Constant_376.991118430775_75d3f/1 -> Product_0c19c/1
  Product_c7c72/1 -> Add_49cf9/2
  State_iq_line_3_6_a71b0/1 -> Product_0c19c/2
  Constant_6354.39881559139_a08a5/1 -> Product_c7c72/1
  Product_0c19c/1 -> Add_49cf9/1
  Constant_6354.39881559139_fd121/1 -> Product_cb8fd/1
  State_vd_bus_6_bb3d9/1 -> Product_cb8fd/2
  Add_49cf9/1 -> Subtract_b6367/1
  Product_cb8fd/1 -> Subtract_b6367/2
  Subtract_b6367/1 -> Blockout_d_id_line_3_6_73b84/1

== system case8/AC_1/d_id_line_4_5_block ==
  note: d_id_line_4_5 in case8
      | $376.991118430775\,\mathrm{iq}_{\mathrm{line},4,5}-64.2696492842669\,\mathrm{id}_{\mathrm{line},4,5}+4047.47576732234\,\mathrm{vd}_{\mathrm{bus},4}-4047.47576732234\,\mathrm{vd}_{\mathrm{bus},5}$
      | Automatically generated on 2025-10-31 19:30:32 .
  State_id_line_4_5_4e862 : Inport
  State_iq_line_4_5_c67ae : Inport  Port=2
  State_vd_bus_4_571f1 : Inport  Port=3
  State_vd_bus_5_769c8 : Inport  Port=4
  Add_a3e90 : Sum
  Add_af823 : Sum
  Constant_-64.2696492842669_e23ff : Constant  Value=-64.2696492842669
  Constant_376.991118430775_e0506 : Constant  Value=376.991118430775
  Constant_4047.47576732234_381dc : Constant  Value=4047.47576732234
  Constant_4047.47576732234_fc879 : Constant  Value=4047.47576732234
  Product_2b98b : Product
  Product_8f1df : Product
  Product_b353c : Product
  Product_f44ca : Product
  Subtract_54930 : Sum  Inputs=+-
  Blockout_d_id_line_4_5_60351 : Outport
  wires:
  Constant_-64.2696492842669_e23ff/1 -> Product_f44ca/1
  Product_b353c/1 -> Add_af823/2
  State_id_line_4_5_4e862/1 -> Product_f44ca/2
  Constant_376.991118430775_e0506/1 -> Product_b353c/1
  State_iq_line_4_5_c67ae/1 -> Product_b353c/2
  Product_f44ca/1 -> Add_af823/1
  Constant_4047.47576732234_381dc/1 -> Product_2b98b/1
  State_vd_bus_4_571f1/1 -> Product_2b98b/2
  Add_af823/1 -> Add_a3e90/1
  Product_2b98b/1 -> Add_a3e90/2
  Constant_4047.47576732234_fc879/1 -> Product_8f1df/1
  State_vd_bus_5_769c8/1 -> Product_8f1df/2
  Add_a3e90/1 -> Subtract_54930/1
  Product_8f1df/1 -> Subtract_54930/2
  Subtract_54930/1 -> Blockout_d_id_line_4_5_60351/1

== system case8/AC_1/d_id_line_5_6_block ==
  note: d_id_line_5_6 in case8
      | $376.991118430775\,\mathrm{iq}_{\mathrm{line},5,6}-79.7922150975604\,\mathrm{id}_{\mathrm{line},5,6}+2190.39865055091\,\mathrm{vd}_{\mathrm{bus},5}-2190.39865055091\,\mathrm{vd}_{\mathrm{bus},6}$
      | Automatically generated on 2025-10-31 19:30:33 .
  State_id_line_5_6_cfe92 : Inport
  State_iq_line_5_6_b7968 : Inport  Port=2
  State_vd_bus_5_80849 : Inport  Port=3
  State_vd_bus_6_fecad : Inport  Port=4
  Add_85872 : Sum
  Add_9417c : Sum
  Constant_-79.7922150975604_14f3b : Constant  Value=-79.7922150975604
  Constant_2190.39865055091_0b21a : Constant  Value=2190.39865055091
  Constant_2190.39865055091_6135b : Constant  Value=2190.39865055091
  Constant_376.991118430775_ecd4e : Constant  Value=376.991118430775
  Product_32ea8 : Product
  Product_40e4a : Product
  Product_7abac : Product
  Product_d0b14 : Product
  Subtract_34351 : Sum  Inputs=+-
  Blockout_d_id_line_5_6_a6fd1 : Outport
  wires:
  Constant_-79.7922150975604_14f3b/1 -> Product_40e4a/1
  Product_7abac/1 -> Add_9417c/2
  State_id_line_5_6_cfe92/1 -> Product_40e4a/2
  Constant_376.991118430775_ecd4e/1 -> Product_7abac/1
  Product_40e4a/1 -> Add_9417c/1
  State_iq_line_5_6_b7968/1 -> Product_7abac/2
  Constant_2190.39865055091_6135b/1 -> Product_32ea8/1
  Product_d0b14/1 -> Subtract_34351/2
  State_vd_bus_5_80849/1 -> Product_32ea8/2
  Add_9417c/1 -> Add_85872/1
  Product_32ea8/1 -> Add_85872/2
  Constant_2190.39865055091_0b21a/1 -> Product_d0b14/1
  State_vd_bus_6_fecad/1 -> Product_d0b14/2
  Add_85872/1 -> Subtract_34351/1
  Subtract_34351/1 -> Blockout_d_id_line_5_6_a6fd1/1

== system case8/AC_1/d_id_line_6_7_block ==
  note: d_id_line_6_7 in case8
      | $376.991118430775\,\mathrm{iq}_{\mathrm{line},6,7}-41.0611648205039\,\mathrm{id}_{\mathrm{line},6,7}+3694.12470827039\,\mathrm{vd}_{\mathrm{bus},6}-3694.12470827039\,\mathrm{vd}_{\mathrm{bus},7}$
      | Automatically generated on 2025-10-31 19:30:35 .
  State_id_line_6_7_0b02a : Inport
  State_iq_line_6_7_677a1 : Inport  Port=2
  State_vd_bus_6_ab512 : Inport  Port=3
  State_vd_bus_7_c4833 : Inport  Port=4
  Add_6e8c6 : Sum
  Add_9284d : Sum
  Constant_-41.0611648205039_5f055 : Constant  Value=-41.0611648205039
  Constant_3694.12470827039_4d5d0 : Constant  Value=3694.12470827039
  Constant_3694.12470827039_5813e : Constant  Value=3694.12470827039
  Constant_376.991118430775_7f6e1 : Constant  Value=376.991118430775
  Product_60d2e : Product
  Product_85c6e : Product
  Product_bd6c1 : Product
  Product_ff634 : Product
  Subtract_3aec1 : Sum  Inputs=+-
  Blockout_d_id_line_6_7_39847 : Outport
  wires:
  Constant_-41.0611648205039_5f055/1 -> Product_bd6c1/1
  Product_ff634/1 -> Add_6e8c6/2
  State_id_line_6_7_0b02a/1 -> Product_bd6c1/2
  Constant_376.991118430775_7f6e1/1 -> Product_ff634/1
  State_iq_line_6_7_677a1/1 -> Product_ff634/2
  Product_bd6c1/1 -> Add_6e8c6/1
  Constant_3694.12470827039_5813e/1 -> Product_60d2e/1
  State_vd_bus_6_ab512/1 -> Product_60d2e/2
  Add_6e8c6/1 -> Add_9284d/1
  Product_60d2e/1 -> Add_9284d/2
  Constant_3694.12470827039_4d5d0/1 -> Product_85c6e/1
  State_vd_bus_7_c4833/1 -> Product_85c6e/2
  Add_9284d/1 -> Subtract_3aec1/1
  Product_85c6e/1 -> Subtract_3aec1/2
  Subtract_3aec1/1 -> Blockout_d_id_line_6_7_39847/1

== system case8/AC_1/d_id_line_7_8_block ==
  note: d_id_line_7_8 in case8
      | $376.991118430775\,\mathrm{iq}_{\mathrm{line},7,8}-41.0611648205039\,\mathrm{id}_{\mathrm{line},7,8}+5171.77459157855\,\mathrm{vd}_{\mathrm{bus},7}-5171.77459157855\,\mathrm{vd}_{\mathrm{bus},8}$
      | Automatically generated on 2025-10-31 19:30:36 .
  State_id_line_7_8_aae09 : Inport
  State_iq_line_7_8_58fab : Inport  Port=2
  State_vd_bus_7_87876 : Inport  Port=3
  State_vd_bus_8_80ba0 : Inport  Port=4
  Add_1328a : Sum
  Add_8a609 : Sum
  Constant_-41.0611648205039_e316e : Constant  Value=-41.0611648205039
  Constant_376.991118430775_38298 : Constant  Value=376.991118430775
  Constant_5171.77459157855_2a9e1 : Constant  Value=5171.77459157855
  Constant_5171.77459157855_9f72e : Constant  Value=5171.77459157855
  Product_0e083 : Product
  Product_a08b6 : Product
  Product_f183d : Product
  Product_f38fa : Product
  Subtract_2e735 : Sum  Inputs=+-
  Blockout_d_id_line_7_8_fdb38 : Outport
  wires:
  Constant_-41.0611648205039_e316e/1 -> Product_f38fa/1
  Product_0e083/1 -> Add_1328a/2
  State_id_line_7_8_aae09/1 -> Product_f38fa/2
  Constant_376.991118430775_38298/1 -> Product_0e083/1
  Product_f38fa/1 -> Add_1328a/1
  State_iq_line_7_8_58fab/1 -> Product_0e083/2
  Constant_5171.77459157855_2a9e1/1 -> Product_f183d/1
  State_vd_bus_7_87876/1 -> Product_f183d/2
  Add_1328a/1 -> Add_8a609/1
  Product_f183d/1 -> Add_8a609/2
  Constant_5171.77459157855_9f72e/1 -> Product_a08b6/1
  State_vd_bus_8_80ba0/1 -> Product_a08b6/2
  Add_8a609/1 -> Subtract_2e735/1
  Product_a08b6/1 -> Subtract_2e735/2
  Subtract_2e735/1 -> Blockout_d_id_line_7_8_fdb38/1

== system case8/AC_1/d_id_line_8_2_block ==
  note: d_id_line_8_2 in case8
      | $376.991118430775\,\mathrm{iq}_{\mathrm{line},8,2}-5957.88432949849\,\mathrm{vd}_{\mathrm{bus},2}+5957.88432949849\,\mathrm{vd}_{\mathrm{bus},8}$
      | Automatically generated on 2025-10-31 19:30:36 .
  State_iq_line_8_2_fcff2 : Inport
  State_vd_bus_2_dc4b2 : Inport  Port=2
  State_vd_bus_8_4b57f : Inport  Port=3
  Add_79b92 : Sum
  Constant_376.991118430775_abf63 : Constant  Value=376.991118430775
  Constant_5957.88432949849_88782 : Constant  Value=5957.88432949849
  Constant_5957.88432949849_f130e : Constant  Value=5957.88432949849
  Product_24775 : Product
  Product_278a7 : Product
  Product_34a01 : Product
  Subtract_b11ac : Sum  Inputs=+-
  Blockout_d_id_line_8_2_3fcd8 : Outport
  wires:
  State_vd_bus_2_dc4b2/1 -> Product_278a7/2
  Constant_376.991118430775_abf63/1 -> Product_24775/1
  Product_278a7/1 -> Subtract_b11ac/2
  State_iq_line_8_2_fcff2/1 -> Product_24775/2
  Constant_5957.88432949849_f130e/1 -> Product_278a7/1
  Product_24775/1 -> Subtract_b11ac/1
  Constant_5957.88432949849_88782/1 -> Product_34a01/1
  State_vd_bus_8_4b57f/1 -> Product_34a01/2
  Subtract_b11ac/1 -> Add_79b92/1
  Product_34a01/1 -> Add_79b92/2
  Add_79b92/1 -> Blockout_d_id_line_8_2_3fcd8/1

== system case8/AC_1/d_id_line_8_9_block ==
  note: d_id_line_8_9 in case8
      | $376.991118430775\,\mathrm{iq}_{\mathrm{line},8,9}-69.1303790620686\,\mathrm{id}_{\mathrm{line},8,9}+2312.84329561277\,\mathrm{vd}_{\mathrm{bus},8}-2312.84329561277\,\mathrm{vd}_{\mathrm{bus},9}$
      | Automatically generated on 2025-10-31 19:30:37 .
  State_id_line_8_9_733fd : Inport
  State_iq_line_8_9_1c9ba : Inport  Port=2
  State_vd_bus_8_052a5 : Inport  Port=3
  State_vd_bus_9_27604 : Inport  Port=4
  Add_21971 : Sum
  Add_4788f : Sum
  Constant_-69.1303790620686_d9474 : Constant  Value=-69.1303790620686
  Constant_2312.84329561277_1f7df : Constant  Value=2312.84329561277
  Constant_2312.84329561277_8742a : Constant  Value=2312.84329561277
  Constant_376.991118430775_dc35f : Constant  Value=376.991118430775
  Product_0b5c0 : Product
  Product_3214a : Product
  Product_79115 : Product
  Product_7ed52 : Product
  Subtract_c2fb4 : Sum  Inputs=+-
  Blockout_d_id_line_8_9_aecdd : Outport
  wires:
  Constant_-69.1303790620686_d9474/1 -> Product_3214a/1
  Product_7ed52/1 -> Add_21971/2
  State_id_line_8_9_733fd/1 -> Product_3214a/2
  Constant_376.991118430775_dc35f/1 -> Product_7ed52/1
  State_iq_line_8_9_1c9ba/1 -> Product_7ed52/2
  Product_3214a/1 -> Add_21971/1
  Constant_2312.84329561277_8742a/1 -> Product_79115/1
  State_vd_bus_8_052a5/1 -> Product_79115/2
  Add_21971/1 -> Add_4788f/1
  Product_79115/1 -> Add_4788f/2
  Constant_2312.84329561277_1f7df/1 -> Product_0b5c0/1
  State_vd_bus_9_27604/1 -> Product_0b5c0/2
  Add_4788f/1 -> Subtract_c2fb4/1
  Product_0b5c0/1 -> Subtract_c2fb4/2
  Subtract_c2fb4/1 -> Blockout_d_id_line_8_9_aecdd/1

== system case8/AC_1/d_id_line_9_4_block ==
  note: d_id_line_9_4 in case8
      | $376.991118430775\,\mathrm{iq}_{\mathrm{line},9,4}-40.9190846654156\,\mathrm{id}_{\mathrm{line},9,4}-4380.79730110183\,\mathrm{vd}_{\mathrm{bus},4}+4380.79730110183\,\mathrm{vd}_{\mathrm{bus},9}$
      | Automatically generated on 2025-10-31 19:30:38 .
  State_id_line_9_4_843c0 : Inport
  State_iq_line_9_4_373f8 : Inport  Port=2
  State_vd_bus_4_5fcff : Inport  Port=3
  State_vd_bus_9_877a7 : Inport  Port=4
  Add_6f145 : Sum
  Add_bcaea : Sum
  Constant_-40.9190846654156_f2298 : Constant  Value=-40.9190846654156
  Constant_376.991118430775_a9965 : Constant  Value=376.991118430775
  Constant_4380.79730110183_0afd0 : Constant  Value=4380.79730110183
  Constant_4380.79730110183_5c4f5 : Constant  Value=4380.79730110183
  Product_70297 : Product
  Product_abbd2 : Product
  Product_c4a9a : Product
  Product_dbbce : Product
  Subtract_4d65f : Sum  Inputs=+-
  Blockout_d_id_line_9_4_fd769 : Outport
  wires:
  Constant_-40.9190846654156_f2298/1 -> Product_c4a9a/1
  Product_70297/1 -> Add_6f145/2
  State_id_line_9_4_843c0/1 -> Product_c4a9a/2
  Constant_376.991118430775_a9965/1 -> Product_70297/1
  Product_c4a9a/1 -> Add_6f145/1
  State_iq_line_9_4_373f8/1 -> Product_70297/2
  Constant_4380.79730110183_5c4f5/1 -> Product_abbd2/1
  State_vd_bus_4_5fcff/1 -> Product_abbd2/2
  Add_6f145/1 -> Subtract_4d65f/1
  Product_abbd2/1 -> Subtract_4d65f/2
  Constant_4380.79730110183_0afd0/1 -> Product_dbbce/1
  Subtract_4d65f/1 -> Add_bcaea/1
  State_vd_bus_9_877a7/1 -> Product_dbbce/2
  Product_dbbce/1 -> Add_bcaea/2
  Add_bcaea/1 -> Blockout_d_id_line_9_4_fd769/1

== system case8/AC_1/d_id_load_5_block ==
  note: d_id_load_5 in case8
      | $376.991118430775\,\mathrm{iq}_{\mathrm{load},5}-1243.06404152488\,\mathrm{id}_{\mathrm{load},5}+1255.7149080224\,\mathrm{vd}_{\mathrm{bus},5}$
      | Automatically generated on 2025-10-31 19:30:29 .
  State_id_load_5_5bf89 : Inport
  State_iq_load_5_baea8 : Inport  Port=2
  State_vd_bus_5_fd6db : Inport  Port=3
  Add_aae56 : Sum
  Add_f2c35 : Sum
  Constant_-1243.06404152488_a013f : Constant  Value=-1243.06404152488
  Constant_1255.7149080224_79975 : Constant  Value=1255.7149080224
  Constant_376.991118430775_71010 : Constant  Value=376.991118430775
  Product_653db : Product
  Product_d2605 : Product
  Product_dbd5e : Product
  Blockout_d_id_load_5_0b5cb : Outport
  wires:
  Constant_-1243.06404152488_a013f/1 -> Product_d2605/1
  Product_dbd5e/1 -> Add_aae56/2
  State_id_load_5_5bf89/1 -> Product_d2605/2
  Constant_376.991118430775_71010/1 -> Product_dbd5e/1
  Product_653db/1 -> Add_f2c35/2
  State_iq_load_5_baea8/1 -> Product_dbd5e/2
  Product_d2605/1 -> Add_aae56/1
  Constant_1255.7149080224_79975/1 -> Product_653db/1
  State_vd_bus_5_fd6db/1 -> Product_653db/2
  Add_aae56/1 -> Add_f2c35/1
  Add_f2c35/1 -> Blockout_d_id_load_5_0b5cb/1
